simulink model "SimpleEKF_2007a"  (Simulink 6.6)
settings: Solver=FixedStepDiscrete  StartTime=0.0  StopTime=300  FixedStep=0.01  RelTol=1e-3
values from neighbouring files (symbols this model uses):
  initP = diag([ 1 1 1 1e5 1e5 1 1e5 1e5 1e5 ])    [SimpleEKF_init.m.m]
undefined symbols (not defined in the file or in its folder): DiscIntNeverNeededParam, gcbh, hwbcalib_subsystem
libraries: simulink x8, dspmtrx3 x5, dspinverses x1
(part 3 of 9)

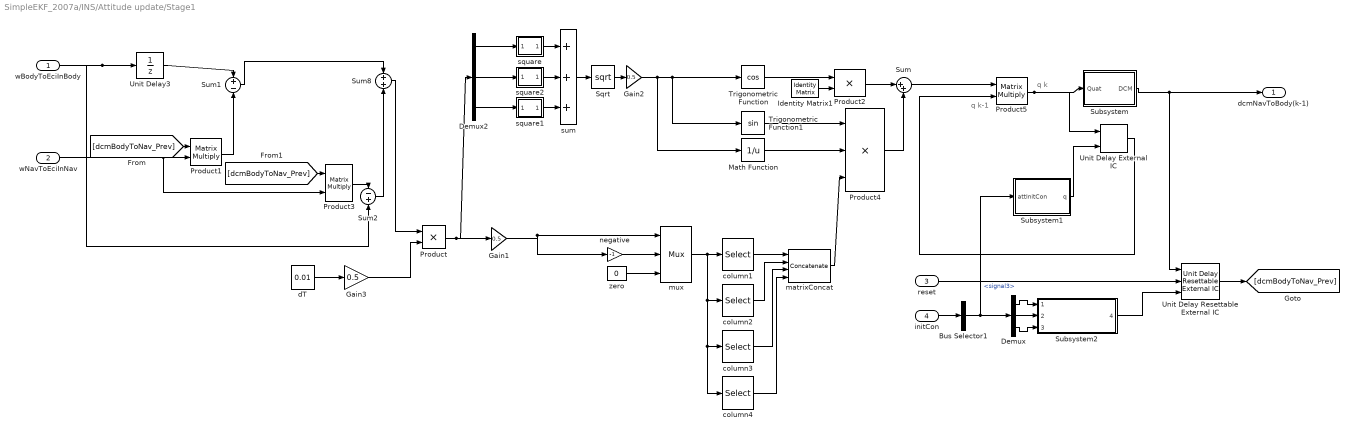
== system SimpleEKF_2007a/INS/Attitude update/Stage1 ==
  note: q k-1
  note: q k
  wBodyToEciInBody : Inport  OutDataType=fixdt(1,16,0)  OutScaling=[]
  wNavToEciInNav : Inport  Port=2  PortDimensions=3  SampleTime=0.01  OutDataType=fixdt(1,16,0)  OutScaling=[]
  reset : Inport  Port=3  PortDimensions=1  SampleTime=0.01  OutDataType=fixdt(1,16,0)  OutScaling=[]
  initCon : Inport  Port=4  OutDataType=fixdt(1,16,0)  OutScaling=[]
  Bus Selector1 : BusSelector  OutputSignals=signal3
  Demux : Demux  Outputs=3
  Demux2 : Demux  Outputs=3
  Gain1 : Gain  Gain=0.5  ParameterDataType=fixdt(1,16,0)  ParameterScaling=[]  OutDataType=fixdt(1,16,0)  OutScaling=[]  SampleTime=0.01
  Gain2 : Gain  Gain=0.5  ParameterDataType=fixdt(1,16,0)  ParameterScaling=[]  OutDataType=fixdt(1,16,0)  OutScaling=[]  SampleTime=0.01
  Gain3 : Gain  Gain=0.5  ParameterDataType=fixdt(1,16,0)  ParameterScaling=[]  OutDataType=fixdt(1,16,0)  OutScaling=[]  SampleTime=0.01
  Identity Matrix1 : dspmtrx3/Identity Matrix  Inherit=off  N=4  Ts=0.01  dataType=double  isSigned=on  wordLen=16  udDataType=sfix(16)  fracBitsMode=Best precision  numFracBits=15
  Math Function : Math  Operator=reciprocal  SampleTime=0.01  OutDataType=fixdt(1,16,0)  OutScaling=[]  SaturateOnIntegerOverflow=on
  Product : Product  OutDataType=fixdt(1,16,0)  OutScaling=[]  RndMeth=Zero
  Product1 : Product  Multiplication=Matrix(*)  OutDataType=fixdt(1,16,0)  OutScaling=[]  SampleTime=0.01  RndMeth=Zero
  Product2 : Product  OutDataType=fixdt(1,16,0)  OutScaling=[]  SampleTime=0.01  RndMeth=Zero
  Product3 : Product  Multiplication=Matrix(*)  OutDataType=fixdt(1,16,0)  OutScaling=[]  SampleTime=0.01  RndMeth=Zero
  Product4 : Product  Inputs=3  OutDataType=fixdt(1,16,0)  OutScaling=[]  SampleTime=0.01  RndMeth=Zero
  Product5 : Product  Multiplication=Matrix(*)  OutDataType=fixdt(1,16,0)  OutScaling=[]  SampleTime=0.01  RndMeth=Zero
  Sqrt : Math  Operator=sqrt  OutDataType=fixdt(1,16,0)  OutScaling=[]  SaturateOnIntegerOverflow=on
  Subsystem : Subsystem
  Subsystem1 : Subsystem
  Subsystem2 : Subsystem
  Sum : Sum  Inputs=|++  OutDataType=fixdt(1,16,0)  OutScaling=[]
  Sum1 : Sum  Inputs=+-  OutDataType=fixdt(1,16,0)  OutScaling=[]  SampleTime=0.01
  Sum2 : Sum  Inputs=-+  OutDataType=fixdt(1,16,0)  OutScaling=[]  SampleTime=0.01
  Sum8 : Sum  OutDataType=fixdt(1,16,0)  OutScaling=[]  SampleTime=0.01
  Trigonometric Function : Trigonometry  Operator=cos  SampleTime=0.01
  Trigonometric Function1 : Trigonometry  SampleTime=0.01
  Unit Delay External IC : simulink/Additional Math & Discrete/Additional Discrete/Unit Delay External IC  SystemSampleTime=-1  tsamp=-1
  Unit Delay Resettable External IC : simulink/Additional Math & Discrete/Additional Discrete/Unit Delay Resettable External IC  SystemSampleTime=-1  tsamp=0.01
  Unit Delay3 : UnitDelay  X0=[0 0 0.]  SampleTime=0.01
  column1 : Selector  Tag=MBDLibrary v2007b.1  IndexOptions=Index vector (dialog)  Indices=[7 1 2 3]  OutputSizes=1  InputPortWidth=7  mask(Mux Selector (MBDLibrary)){InputPortWidth_mbdlib=7, Indices_mbdlib=[7 1 2 3]}
      mask prompts: InputPortWidth_mbdlib "Input Port Width"; Indices_mbdlib "Output Indices"
      mask help: Changes the order of the inputs.
      settings: OpenFcn=|
      | if exist('mbdlib_dialog')
      |    mbdlib_dialog(gcb,'open')
      | else
      |    open_system(gcb, 'mask')
      | end
      settings: CloseFcn=|
      | if exist('mbdlib_selector')
      |    mbdlib_selector(gcb)
      | end
      mask Help: The SELECTOR block is a MULTIPLEXED SELECTOR block, used to change the input/output order of a multiplexed data stream.
      mask Display:
      | port_label('input', 1,'[7]')
      | text(1.0,0.875,'7', 'horizontalAlignment', 'right')
      | text(1.0,0.625,'1', 'horizontalAlignment', 'right')
      | text(1.0,0.375,'2', 'horizontalAlignment', 'right')
      | text(1.0,0.125,'3', 'horizontalAlignment', 'right')
  column2 : Selector  Tag=MBDLibrary v2007b.1  IndexOptions=Index vector (dialog)  Indices=[4 7 6 2]  OutputSizes=1  InputPortWidth=7  mask(Mux Selector (MBDLibrary)){InputPortWidth_mbdlib=7, Indices_mbdlib=[4 7 6 2]}
      mask prompts: InputPortWidth_mbdlib "Input Port Width"; Indices_mbdlib "Output Indices"
      mask help: Changes the order of the inputs.
      settings: OpenFcn=|
      | if exist('mbdlib_dialog')
      |    mbdlib_dialog(gcb,'open')
      | else
      |    open_system(gcb, 'mask')
      | end
      settings: CloseFcn=|
      | if exist('mbdlib_selector')
      |    mbdlib_selector(gcb)
      | end
      mask Help: The SELECTOR block is a MULTIPLEXED SELECTOR block, used to change the input/output order of a multiplexed data stream.
      mask Display:
      | port_label('input', 1,'[7]')
      | text(1.0,0.875,'4', 'horizontalAlignment', 'right')
      | text(1.0,0.625,'7', 'horizontalAlignment', 'right')
      | text(1.0,0.375,'6', 'horizontalAlignment', 'right')
      | text(1.0,0.125,'2', 'horizontalAlignment', 'right')
  column3 : Selector  Tag=MBDLibrary v2007b.1  IndexOptions=Index vector (dialog)  Indices=[5 3 7 4]  OutputSizes=1  InputPortWidth=7  mask(Mux Selector (MBDLibrary)){InputPortWidth_mbdlib=7, Indices_mbdlib=[5 3 7 4]}
      mask prompts: InputPortWidth_mbdlib "Input Port Width"; Indices_mbdlib "Output Indices"
      mask help: Changes the order of the inputs.
      settings: OpenFcn=|
      | if exist('mbdlib_dialog')
      |    mbdlib_dialog(gcb,'open')
      | else
      |    open_system(gcb, 'mask')
      | end
      settings: CloseFcn=|
      | if exist('mbdlib_selector')
      |    mbdlib_selector(gcb)
      | end
      mask Help: The SELECTOR block is a MULTIPLEXED SELECTOR block, used to change the input/output order of a multiplexed data stream.
      mask Display:
      | port_label('input', 1,'[7]')
      | text(1.0,0.875,'5', 'horizontalAlignment', 'right')
      | text(1.0,0.625,'3', 'horizontalAlignment', 'right')
      | text(1.0,0.375,'7', 'horizontalAlignment', 'right')
      | text(1.0,0.125,'4', 'horizontalAlignment', 'right')
  column4 : Selector  Tag=MBDLibrary v2007b.1  IndexOptions=Index vector (dialog)  Indices=[6 5 1 7]  OutputSizes=1  InputPortWidth=7  mask(Mux Selector (MBDLibrary)){InputPortWidth_mbdlib=7, Indices_mbdlib=[6 5 1 7]}
      mask prompts: InputPortWidth_mbdlib "Input Port Width"; Indices_mbdlib "Output Indices"
      mask help: Changes the order of the inputs.
      settings: OpenFcn=|
      | if exist('mbdlib_dialog')
      |    mbdlib_dialog(gcb,'open')
      | else
      |    open_system(gcb, 'mask')
      | end
      settings: CloseFcn=|
      | if exist('mbdlib_selector')
      |    mbdlib_selector(gcb)
      | end
      mask Help: The SELECTOR block is a MULTIPLEXED SELECTOR block, used to change the input/output order of a multiplexed data stream.
      mask Display:
      | port_label('input', 1,'[7]')
      | text(1.0,0.875,'6', 'horizontalAlignment', 'right')
      | text(1.0,0.625,'5', 'horizontalAlignment', 'right')
      | text(1.0,0.375,'1', 'horizontalAlignment', 'right')
      | text(1.0,0.125,'7', 'horizontalAlignment', 'right')
  dT : Constant  Value=0.01  OutDataType=fixdt(1,16,0)  OutScaling=[]
  matrixConcat : Concatenate  Tag=MBDLibrary v2007b.1  NumInputs=4  Mode=Multidimensional array  ConcatenateDimension=2  mask(Matrix Concat (MBDLibrary)){concatDim=Horizontal, numInputs_mbdlib=4}
      mask prompts: concatDim "Type of Concatenate"; numInputs_mbdlib "Number of Inputs"
      mask help: Concatenate input signals of the same data type to create a contiguous output signal.
      settings: OpenFcn=|
      | if exist('mbdlib_dialog')
      |    mbdlib_dialog(gcb,'open')
      | else
      |    open_system(gcb, 'mask')
      | end
      settings: CloseFcn=|
      | if exist('mbdlib_matrixConcatenate')
      |    mbdlib_matrixConcatenate(gcb, 'mask')
      | end
      mask Help:
      | The MATRIX CONCAT block concatenates input signals from the dame data type and creates a contigouos output matrix.
      | In vector mode, all input signals must be either vectors or one-row [1xM] matrices or one-column [Mx1] matrices or a combination of vectors and either one-row matrices or one-column matrices. The output is a vector if all inputs are vectors. The output is a one-row or one-column matrix if any of the inputs are one-row or one-column matrices respectively.
      | 
      | Matrix mode treats vector inputs as one-column matrices. The output is always a matrix.
      mask StyleString: popup(Vertical|Horizontal),edit
      mask Display:
      | plot([0.1 0.3 0.3 0.1 0.1], [0.1 0.1 0.9 0.9 0.1])
      | plot([0.4 0.6 0.6 0.4 0.4], [0.1 0.1 0.9 0.9 0.1])
      | plot([0.7 0.9 0.9 0.7 0.7], [0.1 0.1 0.9 0.9 0.1])
  mux : Mux  Tag=MBDLibrary v2007b.1  Inputs=3  mask(Mux (MBDLibrary)){Inputs_mbdlib=3}
      mask prompts: Inputs_mbdlib "Number of Inputs"
      mask help: Converts multipule inputs to a vector.
      settings: OpenFcn=|
      | if exist('mbdlib_dialog')
      |    mbdlib_dialog(gcb,'open')
      | else
      |    open_system(gcb, 'mask')
      | end
      mask Help: The MUX block provides a vector output to the model for separate inputs.  The output order will correspond to the input order (from the first input at the top of the block to the last input at the bottom of the block).
  negative : Gain  Tag=MBDLibrary v2007b.1  Gain=-1  ParameterDataType=fixdt(1,16,0)  ParameterScaling=[]  OutDataType=fixdt(1,16,0)  OutScaling=[]  RndMeth=Zero  mask(Gain (MBDLibrary)){gain_mbdlib=-1}
      mask prompts: gain_mbdlib "Gain"
      mask help: Multiplies the input by the gain.
      settings: OpenFcn=|
      | if exist('mbdlib_dialog')
      |    mbdlib_dialog(gcb,'open')
      | else
      |    open_system(gcb, 'mask')
      | end
      mask Help: The GAIN block multiplies the input by the gain value.  This block may accept any data types other than boolean.  The user must take care to not use a non-integer gain for int32/uint32 inputs.
      mask Display: disp([get_param(gcb, 'Gain') 'x'])
  square : Subsystem  Tag=MBDLibrary v2007b.1
      settings: OpenFcn=|
      | if exist('mbdlib_dialog')
      |    mbdlib_dialog(gcb,'open')
      | else
      |    open_system(gcb, 'mask')
      | end
      mask Type: Square (MBDLibrary)
      mask Description: Squares the input.
      mask Help: file:///c:\Program Files\MATLAB\R2007b\toolbox\Guidance_and_Navigation_Global\help_files\GeneralUtilities\MBDLibrary\mathfunctions\square.html
      mask Display: disp('x^2', 'texmode', 'on')
  square1 : Subsystem  Tag=MBDLibrary v2007b.1
      settings: OpenFcn=|
      | if exist('mbdlib_dialog')
      |    mbdlib_dialog(gcb,'open')
      | else
      |    open_system(gcb, 'mask')
      | end
      mask Type: Square (MBDLibrary)
      mask Description: Squares the input.
      mask Help: file:///c:\Program Files\MATLAB\R2007b\toolbox\Guidance_and_Navigation_Global\help_files\GeneralUtilities\MBDLibrary\mathfunctions\square.html
      mask Display: disp('x^2', 'texmode', 'on')
  square2 : Subsystem  Tag=MBDLibrary v2007b.1
      settings: OpenFcn=|
      | if exist('mbdlib_dialog')
      |    mbdlib_dialog(gcb,'open')
      | else
      |    open_system(gcb, 'mask')
      | end
      mask Type: Square (MBDLibrary)
      mask Description: Squares the input.
      mask Help: file:///c:\Program Files\MATLAB\R2007b\toolbox\Guidance_and_Navigation_Global\help_files\GeneralUtilities\MBDLibrary\mathfunctions\square.html
      mask Display: disp('x^2', 'texmode', 'on')
  sum : Sum  Tag=MBDLibrary v2007b.1  Inputs=+++  OutDataType=fixdt(1,16,0)  OutScaling=[]  RndMeth=Zero  InputSameDT=on  mask(Sum (MBDLibrary)){inputs_mbdlib=+++}
      mask prompts: inputs_mbdlib "List of signs"
      mask help: Adds values together.
      settings: OpenFcn=|
      | if exist('mbdlib_dialog')
      |    mbdlib_dialog(gcb,'open')
      | else
      |    open_system(gcb, 'mask')
      | end
      mask Help: file:///c:\Program Files\MATLAB\R2007b\toolbox\Guidance_and_Navigation_Global\help_files\GeneralUtilities\MBDLibrary\mathfunctions\sum.html
  zero : Constant  Tag=MBDLibrary v2007b.1  Value=0  VectorParams1D=off  OutDataType=fixdt(1,16,0)  OutScaling=[]  mask(Constant (MBDLibrary)){Value_mbdlib=0, OutDataTypeMode_mbdlib=double}
      mask prompts: Value_mbdlib "Constant"; OutDataTypeMode_mbdlib "Data Type"
      mask help: Outputs a constant value
      settings: AttributesFormatString={%<OutDataTypeMode>}
      settings: OpenFcn=|
      | if exist('mbdlib_dialog')
      |    mbdlib_dialog(gcb,'open')
      | else
      |    open_system(gcb, 'mask')
      | end
      settings: CloseFcn=|
      | if exist('mbdlib_dialog')
      |    mbdlib_constant(gcb)
      | end
      mask Help: The CONSTANT block outputs a constant value to the system.
      mask StyleString: edit,popup(double|single|boolean|int32|uint32)
  dcmNavToBody(k-1) : Outport  OutDataType=fixdt(1,16,0)  OutScaling=[]
  wires:
  wBodyToEciInBody/1 -> Sum2/2, Unit Delay3/1
  wNavToEciInNav/1 -> Product1/2, Product3/2
  Demux2/3 -> square1/1(squareLibIn)
  Subsystem/1(DCM) -> dcmNavToBody(k-1)/1, Unit Delay Resettable External IC/1
  Demux2/2 -> square2/1(squareLibIn)
  Unit Delay External IC/1 -> Product5/2
  Product5/1 -> Unit Delay External IC/1, Subsystem/1(Quat)
  Sum/1 -> Product5/1
  Product4/1 -> Sum/2
  Product2/1 -> Sum/1
  Identity Matrix1/1 -> Product2/2
  Trigonometric Function/1 -> Product2/1
  Gain2/1 -> Math Function/1, Trigonometric Function/1, Trigonometric Function1/1
  Sqrt/1 -> Gain2/1
  sum/1 -> Sqrt/1
  square1/1(squareLibOut) -> sum/3
  square2/1(squareLibOut) -> sum/2
  square/1(squareLibOut) -> sum/1
  Demux2/1 -> square/1(squareLibIn)
  column4/1 -> matrixConcat/4
  Gain1/1 -> mux/1, negative/1
  mux/1 -> column2/1, column3/1, column4/1, column1/1
  column1/1 -> matrixConcat/1
  column2/1 -> matrixConcat/2
  column3/1 -> matrixConcat/3
  negative/1 -> mux/2
  zero/1 -> mux/3
  Sum1/1 -> Sum8/1
  Sum2/1 -> Sum8/2
  Product3/1 -> Sum2/1
  Unit Delay3/1 -> Sum1/1
  Product1/1 -> Sum1/2
  dT/1 -> Gain3/1
  Sum8/1 -> Product/1
  Gain3/1 -> Product/2
  Product/1 -> Gain1/1, Demux2/1
  [dcmBodyToNav_Prev] -> Product1/1
  [dcmBodyToNav_Prev] -> Product3/1
  Trigonometric Function1/1 -> Product4/1
  Math Function/1 -> Product4/2
  matrixConcat/1 -> Product4/3
  Subsystem1/1(q) -> Unit Delay External IC/2
  reset/1 -> Unit Delay Resettable External IC/2
  initCon/1 -> Bus Selector1/1
  Bus Selector1/1 -> Demux/1, Subsystem1/1(attInitCon)  "<signal3>"
  Demux/1 -> Subsystem2/1(1)
  Demux/2 -> Subsystem2/2(2)
  Demux/3 -> Subsystem2/3(3)
  Unit Delay Resettable External IC/1 -> [dcmBodyToNav_Prev]
  Subsystem2/1(4) -> Unit Delay Resettable External IC/3

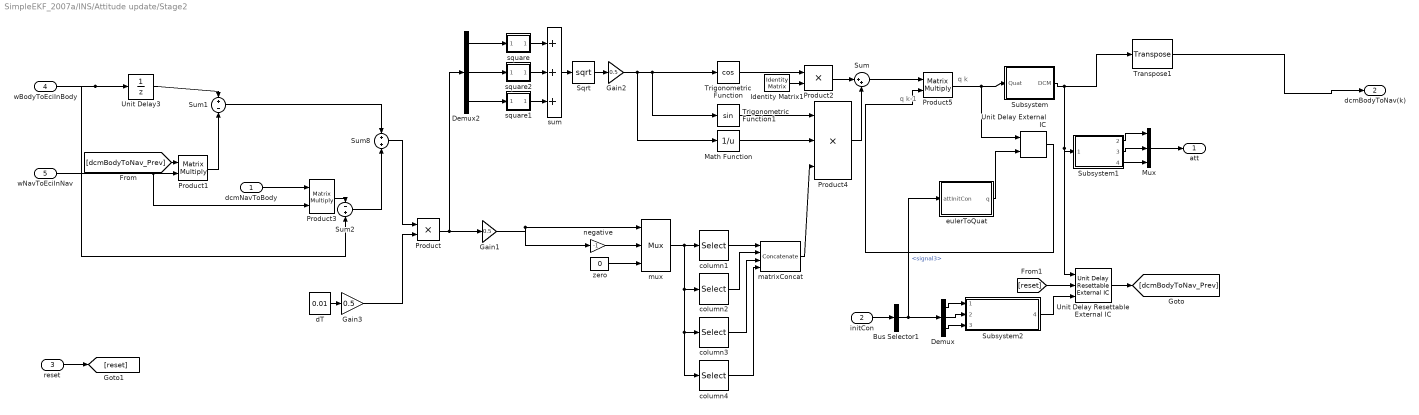
== system SimpleEKF_2007a/INS/Attitude update/Stage2 ==
  note: q k-1
  note: q k
  dcmNavToBody : Inport  PortDimensions=[3,3]  SampleTime=0.01  OutDataType=fixdt(1,16,0)  OutScaling=[]
  initCon : Inport  Port=2  OutDataType=fixdt(1,16,0)  OutScaling=[]
  reset : Inport  Port=3  PortDimensions=1  SampleTime=0.01  OutDataType=fixdt(1,16,0)  OutScaling=[]
  wBodyToEciInBody : Inport  Port=4  PortDimensions=3  SampleTime=0.01  OutDataType=fixdt(1,16,0)  OutScaling=[]
  wNavToEciInNav : Inport  Port=5  PortDimensions=3  SampleTime=0.01  OutDataType=fixdt(1,16,0)  OutScaling=[]
  Bus Selector1 : BusSelector  OutputSignals=signal3
  Demux : Demux  Outputs=3
  Demux2 : Demux  Outputs=3
  Gain1 : Gain  Gain=0.5  ParameterDataType=fixdt(1,16,0)  ParameterScaling=[]  OutDataType=fixdt(1,16,0)  OutScaling=[]  SampleTime=0.01
  Gain2 : Gain  Gain=0.5  ParameterDataType=fixdt(1,16,0)  ParameterScaling=[]  OutDataType=fixdt(1,16,0)  OutScaling=[]  SampleTime=0.01
  Gain3 : Gain  Gain=0.5  ParameterDataType=fixdt(1,16,0)  ParameterScaling=[]  OutDataType=fixdt(1,16,0)  OutScaling=[]  SampleTime=0.01
  Identity Matrix1 : dspmtrx3/Identity Matrix  Inherit=off  N=4  Ts=0.01  dataType=double  isSigned=on  wordLen=16  udDataType=sfix(16)  fracBitsMode=Best precision  numFracBits=15
  Math Function : Math  Operator=reciprocal  SampleTime=0.01  OutDataType=fixdt(1,16,0)  OutScaling=[]  SaturateOnIntegerOverflow=on
  Mux : Mux  Inputs=3
  Product : Product  OutDataType=fixdt(1,16,0)  OutScaling=[]  RndMeth=Zero
  Product1 : Product  Multiplication=Matrix(*)  OutDataType=fixdt(1,16,0)  OutScaling=[]  SampleTime=0.01  RndMeth=Zero
  Product2 : Product  OutDataType=fixdt(1,16,0)  OutScaling=[]  SampleTime=0.01  RndMeth=Zero
  Product3 : Product  Multiplication=Matrix(*)  OutDataType=fixdt(1,16,0)  OutScaling=[]  SampleTime=0.01  RndMeth=Zero
  Product4 : Product  Inputs=3  OutDataType=fixdt(1,16,0)  OutScaling=[]  SampleTime=0.01  RndMeth=Zero
  Product5 : Product  Multiplication=Matrix(*)  OutDataType=fixdt(1,16,0)  OutScaling=[]  SampleTime=0.01  RndMeth=Zero
  Sqrt : Math  Operator=sqrt  OutDataType=fixdt(1,16,0)  OutScaling=[]  SaturateOnIntegerOverflow=on
  Subsystem : Subsystem
  Subsystem1 : Subsystem
  Subsystem2 : Subsystem
  Sum : Sum  Inputs=|++  OutDataType=fixdt(1,16,0)  OutScaling=[]
  Sum1 : Sum  Inputs=+-  OutDataType=fixdt(1,16,0)  OutScaling=[]  SampleTime=0.01
  Sum2 : Sum  Inputs=-+  OutDataType=fixdt(1,16,0)  OutScaling=[]  SampleTime=0.01
  Sum8 : Sum  OutDataType=fixdt(1,16,0)  OutScaling=[]  SampleTime=0.01
  Transpose1 : dspmtrx3/Transpose  SystemSampleTime=-1  Hermitian=off  overflowFlag=off
  Trigonometric Function : Trigonometry  Operator=cos  SampleTime=0.01
  Trigonometric Function1 : Trigonometry  SampleTime=0.01
  Unit Delay External IC : simulink/Additional Math & Discrete/Additional Discrete/Unit Delay External IC  SystemSampleTime=-1  tsamp=-1
  Unit Delay Resettable External IC : simulink/Additional Math & Discrete/Additional Discrete/Unit Delay Resettable External IC  SystemSampleTime=-1  tsamp=0.01
  Unit Delay3 : UnitDelay  X0=[0 0 0]  SampleTime=0.01
  column1 : Selector  Tag=MBDLibrary v2007b.1  IndexOptions=Index vector (dialog)  Indices=[7 1 2 3]  OutputSizes=1  InputPortWidth=7  mask(Mux Selector (MBDLibrary)){InputPortWidth_mbdlib=7, Indices_mbdlib=[7 1 2 3]}
      mask prompts: InputPortWidth_mbdlib "Input Port Width"; Indices_mbdlib "Output Indices"
      mask help: Changes the order of the inputs.
      settings: OpenFcn=|
      | if exist('mbdlib_dialog')
      |    mbdlib_dialog(gcb,'open')
      | else
      |    open_system(gcb, 'mask')
      | end
      settings: CloseFcn=|
      | if exist('mbdlib_selector')
      |    mbdlib_selector(gcb)
      | end
      mask Help: The SELECTOR block is a MULTIPLEXED SELECTOR block, used to change the input/output order of a multiplexed data stream.
      mask Display:
      | port_label('input', 1,'[7]')
      | text(1.0,0.875,'7', 'horizontalAlignment', 'right')
      | text(1.0,0.625,'1', 'horizontalAlignment', 'right')
      | text(1.0,0.375,'2', 'horizontalAlignment', 'right')
      | text(1.0,0.125,'3', 'horizontalAlignment', 'right')
  column2 : Selector  Tag=MBDLibrary v2007b.1  IndexOptions=Index vector (dialog)  Indices=[4 7 6 2]  OutputSizes=1  InputPortWidth=7  mask(Mux Selector (MBDLibrary)){InputPortWidth_mbdlib=7, Indices_mbdlib=[4 7 6 2]}
      mask prompts: InputPortWidth_mbdlib "Input Port Width"; Indices_mbdlib "Output Indices"
      mask help: Changes the order of the inputs.
      settings: OpenFcn=|
      | if exist('mbdlib_dialog')
      |    mbdlib_dialog(gcb,'open')
      | else
      |    open_system(gcb, 'mask')
      | end
      settings: CloseFcn=|
      | if exist('mbdlib_selector')
      |    mbdlib_selector(gcb)
      | end
      mask Help: The SELECTOR block is a MULTIPLEXED SELECTOR block, used to change the input/output order of a multiplexed data stream.
      mask Display:
      | port_label('input', 1,'[7]')
      | text(1.0,0.875,'4', 'horizontalAlignment', 'right')
      | text(1.0,0.625,'7', 'horizontalAlignment', 'right')
      | text(1.0,0.375,'6', 'horizontalAlignment', 'right')
      | text(1.0,0.125,'2', 'horizontalAlignment', 'right')
  column3 : Selector  Tag=MBDLibrary v2007b.1  IndexOptions=Index vector (dialog)  Indices=[5 3 7 4]  OutputSizes=1  InputPortWidth=7  mask(Mux Selector (MBDLibrary)){InputPortWidth_mbdlib=7, Indices_mbdlib=[5 3 7 4]}
      mask prompts: InputPortWidth_mbdlib "Input Port Width"; Indices_mbdlib "Output Indices"
      mask help: Changes the order of the inputs.
      settings: OpenFcn=|
      | if exist('mbdlib_dialog')
      |    mbdlib_dialog(gcb,'open')
      | else
      |    open_system(gcb, 'mask')
      | end
      settings: CloseFcn=|
      | if exist('mbdlib_selector')
      |    mbdlib_selector(gcb)
      | end
      mask Help: The SELECTOR block is a MULTIPLEXED SELECTOR block, used to change the input/output order of a multiplexed data stream.
      mask Display:
      | port_label('input', 1,'[7]')
      | text(1.0,0.875,'5', 'horizontalAlignment', 'right')
      | text(1.0,0.625,'3', 'horizontalAlignment', 'right')
      | text(1.0,0.375,'7', 'horizontalAlignment', 'right')
      | text(1.0,0.125,'4', 'horizontalAlignment', 'right')
  column4 : Selector  Tag=MBDLibrary v2007b.1  IndexOptions=Index vector (dialog)  Indices=[6 5 1 7]  OutputSizes=1  InputPortWidth=7  mask(Mux Selector (MBDLibrary)){InputPortWidth_mbdlib=7, Indices_mbdlib=[6 5 1 7]}
      mask prompts: InputPortWidth_mbdlib "Input Port Width"; Indices_mbdlib "Output Indices"
      mask help: Changes the order of the inputs.
      settings: OpenFcn=|
      | if exist('mbdlib_dialog')
      |    mbdlib_dialog(gcb,'open')
      | else
      |    open_system(gcb, 'mask')
      | end
      settings: CloseFcn=|
      | if exist('mbdlib_selector')
      |    mbdlib_selector(gcb)
      | end
      mask Help: The SELECTOR block is a MULTIPLEXED SELECTOR block, used to change the input/output order of a multiplexed data stream.
      mask Display:
      | port_label('input', 1,'[7]')
      | text(1.0,0.875,'6', 'horizontalAlignment', 'right')
      | text(1.0,0.625,'5', 'horizontalAlignment', 'right')
      | text(1.0,0.375,'1', 'horizontalAlignment', 'right')
      | text(1.0,0.125,'7', 'horizontalAlignment', 'right')
  dT : Constant  Value=0.01  OutDataType=fixdt(1,16,0)  OutScaling=[]
  eulerToQuat : Subsystem
  matrixConcat : Concatenate  Tag=MBDLibrary v2007b.1  NumInputs=4  Mode=Multidimensional array  ConcatenateDimension=2  mask(Matrix Concat (MBDLibrary)){concatDim=Horizontal, numInputs_mbdlib=4}
      mask prompts: concatDim "Type of Concatenate"; numInputs_mbdlib "Number of Inputs"
      mask help: Concatenate input signals of the same data type to create a contiguous output signal.
      settings: OpenFcn=|
      | if exist('mbdlib_dialog')
      |    mbdlib_dialog(gcb,'open')
      | else
      |    open_system(gcb, 'mask')
      | end
      settings: CloseFcn=|
      | if exist('mbdlib_matrixConcatenate')
      |    mbdlib_matrixConcatenate(gcb, 'mask')
      | end
      mask Help:
      | The MATRIX CONCAT block concatenates input signals from the dame data type and creates a contigouos output matrix.
      | In vector mode, all input signals must be either vectors or one-row [1xM] matrices or one-column [Mx1] matrices or a combination of vectors and either one-row matrices or one-column matrices. The output is a vector if all inputs are vectors. The output is a one-row or one-column matrix if any of the inputs are one-row or one-column matrices respectively.
      | 
      | Matrix mode treats vector inputs as one-column matrices. The output is always a matrix.
      mask StyleString: popup(Vertical|Horizontal),edit
      mask Display:
      | plot([0.1 0.3 0.3 0.1 0.1], [0.1 0.1 0.9 0.9 0.1])
      | plot([0.4 0.6 0.6 0.4 0.4], [0.1 0.1 0.9 0.9 0.1])
      | plot([0.7 0.9 0.9 0.7 0.7], [0.1 0.1 0.9 0.9 0.1])
  mux : Mux  Tag=MBDLibrary v2007b.1  Inputs=3  mask(Mux (MBDLibrary)){Inputs_mbdlib=3}
      mask prompts: Inputs_mbdlib "Number of Inputs"
      mask help: Converts multipule inputs to a vector.
      settings: OpenFcn=|
      | if exist('mbdlib_dialog')
      |    mbdlib_dialog(gcb,'open')
      | else
      |    open_system(gcb, 'mask')
      | end
      mask Help: The MUX block provides a vector output to the model for separate inputs.  The output order will correspond to the input order (from the first input at the top of the block to the last input at the bottom of the block).
  negative : Gain  Tag=MBDLibrary v2007b.1  Gain=-1  ParameterDataType=fixdt(1,16,0)  ParameterScaling=[]  OutDataType=fixdt(1,16,0)  OutScaling=[]  RndMeth=Zero  mask(Gain (MBDLibrary)){gain_mbdlib=-1}
      mask prompts: gain_mbdlib "Gain"
      mask help: Multiplies the input by the gain.
      settings: OpenFcn=|
      | if exist('mbdlib_dialog')
      |    mbdlib_dialog(gcb,'open')
      | else
      |    open_system(gcb, 'mask')
      | end
      mask Help: The GAIN block multiplies the input by the gain value.  This block may accept any data types other than boolean.  The user must take care to not use a non-integer gain for int32/uint32 inputs.
      mask Display: disp([get_param(gcb, 'Gain') 'x'])
  square : Subsystem  Tag=MBDLibrary v2007b.1
      settings: OpenFcn=|
      | if exist('mbdlib_dialog')
      |    mbdlib_dialog(gcb,'open')
      | else
      |    open_system(gcb, 'mask')
      | end
      mask Type: Square (MBDLibrary)
      mask Description: Squares the input.
      mask Help: file:///c:\Program Files\MATLAB\R2007b\toolbox\Guidance_and_Navigation_Global\help_files\GeneralUtilities\MBDLibrary\mathfunctions\square.html
      mask Display: disp('x^2', 'texmode', 'on')
  square1 : Subsystem  Tag=MBDLibrary v2007b.1
      settings: OpenFcn=|
      | if exist('mbdlib_dialog')
      |    mbdlib_dialog(gcb,'open')
      | else
      |    open_system(gcb, 'mask')
      | end
      mask Type: Square (MBDLibrary)
      mask Description: Squares the input.
      mask Help: file:///c:\Program Files\MATLAB\R2007b\toolbox\Guidance_and_Navigation_Global\help_files\GeneralUtilities\MBDLibrary\mathfunctions\square.html
      mask Display: disp('x^2', 'texmode', 'on')
  square2 : Subsystem  Tag=MBDLibrary v2007b.1
      settings: OpenFcn=|
      | if exist('mbdlib_dialog')
      |    mbdlib_dialog(gcb,'open')
      | else
      |    open_system(gcb, 'mask')
      | end
      mask Type: Square (MBDLibrary)
      mask Description: Squares the input.
      mask Help: file:///c:\Program Files\MATLAB\R2007b\toolbox\Guidance_and_Navigation_Global\help_files\GeneralUtilities\MBDLibrary\mathfunctions\square.html
      mask Display: disp('x^2', 'texmode', 'on')
  sum : Sum  Tag=MBDLibrary v2007b.1  Inputs=+++  OutDataType=fixdt(1,16,0)  OutScaling=[]  RndMeth=Zero  InputSameDT=on  mask(Sum (MBDLibrary)){inputs_mbdlib=+++}
      mask prompts: inputs_mbdlib "List of signs"
      mask help: Adds values together.
      settings: OpenFcn=|
      | if exist('mbdlib_dialog')
      |    mbdlib_dialog(gcb,'open')
      | else
      |    open_system(gcb, 'mask')
      | end
      mask Help: file:///c:\Program Files\MATLAB\R2007b\toolbox\Guidance_and_Navigation_Global\help_files\GeneralUtilities\MBDLibrary\mathfunctions\sum.html
  zero : Constant  Tag=MBDLibrary v2007b.1  Value=0  VectorParams1D=off  OutDataType=fixdt(1,16,0)  OutScaling=[]  mask(Constant (MBDLibrary)){Value_mbdlib=0, OutDataTypeMode_mbdlib=double}
      mask prompts: Value_mbdlib "Constant"; OutDataTypeMode_mbdlib "Data Type"
      mask help: Outputs a constant value
      settings: AttributesFormatString={%<OutDataTypeMode>}
      settings: OpenFcn=|
      | if exist('mbdlib_dialog')
      |    mbdlib_dialog(gcb,'open')
      | else
      |    open_system(gcb, 'mask')
      | end
      settings: CloseFcn=|
      | if exist('mbdlib_dialog')
      |    mbdlib_constant(gcb)
      | end
      mask Help: The CONSTANT block outputs a constant value to the system.
      mask StyleString: edit,popup(double|single|boolean|int32|uint32)
  att : Outport  PortDimensions=3  SampleTime=0.01  OutDataType=fixdt(1,16,0)  OutScaling=[]
  dcmBodyToNav(k) : Outport  Port=2  OutDataType=fixdt(1,16,0)  OutScaling=[]
  wires:
  wBodyToEciInBody/1 -> Sum2/2, Unit Delay3/1
  wNavToEciInNav/1 -> Product1/2, Product3/2
  Demux2/3 -> square1/1(squareLibIn)
  Subsystem/1(DCM) -> Unit Delay Resettable External IC/1, Subsystem1/1(1), Transpose1/1
  Demux2/2 -> square2/1(squareLibIn)
  Product5/1 -> Unit Delay External IC/1, Subsystem/1(Quat)
  Sum/1 -> Product5/1
  Product4/1 -> Sum/2
  Product2/1 -> Sum/1
  Identity Matrix1/1 -> Product2/2
  Trigonometric Function/1 -> Product2/1
  Gain2/1 -> Math Function/1, Trigonometric Function/1, Trigonometric Function1/1
  Sqrt/1 -> Gain2/1
  sum/1 -> Sqrt/1
  square1/1(squareLibOut) -> sum/3
  square2/1(squareLibOut) -> sum/2
  square/1(squareLibOut) -> sum/1
  Demux2/1 -> square/1(squareLibIn)
  column4/1 -> matrixConcat/4
  Gain1/1 -> mux/1, negative/1
  mux/1 -> column2/1, column3/1, column4/1, column1/1
  column1/1 -> matrixConcat/1
  column2/1 -> matrixConcat/2
  column3/1 -> matrixConcat/3
  negative/1 -> mux/2
  zero/1 -> mux/3
  Sum1/1 -> Sum8/1
  Sum2/1 -> Sum8/2
  Product3/1 -> Sum2/1
  Unit Delay3/1 -> Sum1/1
  Product1/1 -> Sum1/2
  dT/1 -> Gain3/1
  Sum8/1 -> Product/1
  Gain3/1 -> Product/2
  Product/1 -> Gain1/1, Demux2/1
  [dcmBodyToNav_Prev] -> Product1/1
  Trigonometric Function1/1 -> Product4/1
  Math Function/1 -> Product4/2
  dcmNavToBody/1 -> Product3/1
  Subsystem1/1(2) -> Mux/1
  Subsystem1/2(3) -> Mux/2
  Subsystem1/3(4) -> Mux/3
  matrixConcat/1 -> Product4/3
  Unit Delay Resettable External IC/1 -> [dcmBodyToNav_Prev]
  initCon/1 -> Bus Selector1/1
  Bus Selector1/1 -> Demux/1, eulerToQuat/1(attInitCon)  "<signal3>"
  Demux/1 -> Subsystem2/1(1)
  Demux/2 -> Subsystem2/2(2)
  Demux/3 -> Subsystem2/3(3)
  Unit Delay External IC/1 -> Product5/2
  eulerToQuat/1(q) -> Unit Delay External IC/2
  reset/1 -> [reset]
  [reset] -> Unit Delay Resettable External IC/2
  Subsystem2/1(4) -> Unit Delay Resettable External IC/3
  Transpose1/1 -> dcmBodyToNav(k)/1
  Mux/1 -> att/1

== system SimpleEKF_2007a/INS/Coriolis correction/RM ==
  pos_lat : Inport  PortDimensions=1  SampleTime=0.01  OutDataType=fixdt(1,16,0)  OutScaling=[]
  Constant : Constant  OutDataType=fixdt(1,16,0)  OutScaling=[]
  Constant1 : Constant  Value=1.5  OutDataType=fixdt(1,16,0)  OutScaling=[]
  Math Function : Math  Operator=pow  OutDataType=fixdt(1,16,0)  OutScaling=[]  SaturateOnIntegerOverflow=on
  Product : Product  OutDataType=fixdt(1,16,0)  OutScaling=[]  RndMeth=Zero
  Product1 : Product  OutDataType=fixdt(1,16,0)  OutScaling=[]  RndMeth=Zero
  Sum : Sum  Inputs=|+-  OutDataType=fixdt(1,16,0)  OutScaling=[]
  Sum1 : Sum  Inputs=|+-  OutDataType=fixdt(1,16,0)  OutScaling=[]
  Trigonometric Function : Trigonometry
  constant : Constant  Tag=MBDLibrary v2007b.1  VectorParams1D=off  OutDataType=fixdt(1,16,0)  OutScaling=[]  mask(Constant (MBDLibrary)){Value_mbdlib=1, OutDataTypeMode_mbdlib=double}
      mask prompts: Value_mbdlib "Constant"; OutDataTypeMode_mbdlib "Data Type"
      mask help: Outputs a constant value
      settings: AttributesFormatString={%<OutDataTypeMode>}
      settings: OpenFcn=|
      | if exist('mbdlib_dialog')
      |    mbdlib_dialog(gcb,'open')
      | else
      |    open_system(gcb, 'mask')
      | end
      settings: CloseFcn=|
      | if exist('mbdlib_dialog')
      |    mbdlib_constant(gcb)
      | end
      mask Help: file:///c:\Program Files\MATLAB\R2007b\toolbox\Guidance_and_Navigation_Global\help_files\GeneralUtilities\MBDLibrary\mathfunctions\constant.html
      mask StyleString: edit,popup(double|single|boolean|int32|uint32)
  divide : Product  Tag=MBDLibrary v2007b.1  Inputs=*/  OutDataType=fixdt(1,16,0)  OutScaling=[]  RndMeth=Zero  InputSameDT=on
      settings: OpenFcn=|
      | if exist('mbdlib_dialog')
      |    mbdlib_dialog(gcb,'open')
      | else
      |    open_system(gcb, 'mask')
      | end
      mask Type: Divide (MBDLibrary)
      mask Description: Divides two inputs.
      mask Help: file:///c:\Program Files\MATLAB\R2007b\toolbox\Guidance_and_Navigation_Global\help_files\GeneralUtilities\MBDLibrary\mathfunctions\divide.html
      mask Display:
      | port_label('input',1,'n')
      | port_label('input',2,'d')
      | port_label('output',1,'n/d')
  epsilon : Constant  Value=0.0818191908426  OutDataType=fixdt(1,16,0)  OutScaling=[]
  re : Constant  Value=6378137  OutDataType=fixdt(1,16,0)  OutScaling=[]
  square : Subsystem  Tag=MBDLibrary v2007b.1
      settings: OpenFcn=|
      | if exist('mbdlib_dialog')
      |    mbdlib_dialog(gcb,'open')
      | else
      |    open_system(gcb, 'mask')
      | end
      mask Type: Square (MBDLibrary)
      mask Description: Squares the input.
      mask Help: file:///c:\Program Files\MATLAB\R2007b\toolbox\Guidance_and_Navigation_Global\help_files\GeneralUtilities\MBDLibrary\mathfunctions\square.html
      mask Display: disp('x^2', 'texmode', 'on')
  square1 : Subsystem  Tag=MBDLibrary v2007b.1
      settings: OpenFcn=|
      | if exist('mbdlib_dialog')
      |    mbdlib_dialog(gcb,'open')
      | else
      |    open_system(gcb, 'mask')
      | end
      mask Type: Square (MBDLibrary)
      mask Description: Squares the input.
      mask Help: file:///c:\Program Files\MATLAB\R2007b\toolbox\Guidance_and_Navigation_Global\help_files\GeneralUtilities\MBDLibrary\mathfunctions\square.html
      mask Display: disp('x^2', 'texmode', 'on')
  rm : Outport  PortDimensions=1  SampleTime=0.01  OutDataType=fixdt(1,16,0)  OutScaling=[]
  wires:
  constant/1 -> Sum/1
  epsilon/1 -> square1/1(squareLibIn)
  square1/1(squareLibOut) -> Product/1, Sum1/2
  pos_lat/1 -> Trigonometric Function/1
  Trigonometric Function/1 -> square/1(squareLibIn)
  square/1(squareLibOut) -> Product/2
  Product/1 -> Sum/2
  Sum/1 -> Math Function/1
  divide/1 -> rm/1
  Constant/1 -> Sum1/1
  Constant1/1 -> Math Function/2
  Math Function/1 -> divide/2
  re/1 -> Product1/1
  Sum1/1 -> Product1/2
  Product1/1 -> divide/1

== system SimpleEKF_2007a/INS/Coriolis correction/RN ==
  pos_lat : Inport  PortDimensions=1  SampleTime=0.01  OutDataType=fixdt(1,16,0)  OutScaling=[]
  Product : Product  OutDataType=fixdt(1,16,0)  OutScaling=[]  RndMeth=Zero
  Sqrt : Math  Operator=sqrt  OutDataType=fixdt(1,16,0)  OutScaling=[]  SaturateOnIntegerOverflow=on
  Sum : Sum  Inputs=|+-  OutDataType=fixdt(1,16,0)  OutScaling=[]
  Trigonometric Function : Trigonometry
  constant : Constant  Tag=MBDLibrary v2007b.1  VectorParams1D=off  OutDataType=fixdt(1,16,0)  OutScaling=[]  mask(Constant (MBDLibrary)){Value_mbdlib=1, OutDataTypeMode_mbdlib=double}
      mask prompts: Value_mbdlib "Constant"; OutDataTypeMode_mbdlib "Data Type"
      mask help: Outputs a constant value
      settings: AttributesFormatString={%<OutDataTypeMode>}
      settings: OpenFcn=|
      | if exist('mbdlib_dialog')
      |    mbdlib_dialog(gcb,'open')
      | else
      |    open_system(gcb, 'mask')
      | end
      settings: CloseFcn=|
      | if exist('mbdlib_dialog')
      |    mbdlib_constant(gcb)
      | end
      mask Help: file:///c:\Program Files\MATLAB\R2007b\toolbox\Guidance_and_Navigation_Global\help_files\GeneralUtilities\MBDLibrary\mathfunctions\constant.html
      mask StyleString: edit,popup(double|single|boolean|int32|uint32)
  divide : Product  Tag=MBDLibrary v2007b.1  Inputs=*/  OutDataType=fixdt(1,16,0)  OutScaling=[]  RndMeth=Zero  InputSameDT=on
      settings: OpenFcn=|
      | if exist('mbdlib_dialog')
      |    mbdlib_dialog(gcb,'open')
      | else
      |    open_system(gcb, 'mask')
      | end
      mask Type: Divide (MBDLibrary)
      mask Description: Divides two inputs.
      mask Help: file:///c:\Program Files\MATLAB\R2007b\toolbox\Guidance_and_Navigation_Global\help_files\GeneralUtilities\MBDLibrary\mathfunctions\divide.html
      mask Display:
      | port_label('input',1,'n')
      | port_label('input',2,'d')
      | port_label('output',1,'n/d')
  epsilon : Constant  Value=0.0818191908426  OutDataType=fixdt(1,16,0)  OutScaling=[]
  re : Constant  Value=6378137  OutDataType=fixdt(1,16,0)  OutScaling=[]
  square : Subsystem  Tag=MBDLibrary v2007b.1
      settings: OpenFcn=|
      | if exist('mbdlib_dialog')
      |    mbdlib_dialog(gcb,'open')
      | else
      |    open_system(gcb, 'mask')
      | end
      mask Type: Square (MBDLibrary)
      mask Description: Squares the input.
      mask Help: file:///c:\Program Files\MATLAB\R2007b\toolbox\Guidance_and_Navigation_Global\help_files\GeneralUtilities\MBDLibrary\mathfunctions\square.html
      mask Display: disp('x^2', 'texmode', 'on')
  square1 : Subsystem  Tag=MBDLibrary v2007b.1
      settings: OpenFcn=|
      | if exist('mbdlib_dialog')
      |    mbdlib_dialog(gcb,'open')
      | else
      |    open_system(gcb, 'mask')
      | end
      mask Type: Square (MBDLibrary)
      mask Description: Squares the input.
      mask Help: file:///c:\Program Files\MATLAB\R2007b\toolbox\Guidance_and_Navigation_Global\help_files\GeneralUtilities\MBDLibrary\mathfunctions\square.html
      mask Display: disp('x^2', 'texmode', 'on')
  rn : Outport  PortDimensions=1  SampleTime=0.01  OutDataType=fixdt(1,16,0)  OutScaling=[]
  wires:
  re/1 -> divide/1
  constant/1 -> Sum/1
  epsilon/1 -> square1/1(squareLibIn)
  square1/1(squareLibOut) -> Product/1
  pos_lat/1 -> Trigonometric Function/1
  Trigonometric Function/1 -> square/1(squareLibIn)
  square/1(squareLibOut) -> Product/2
  Product/1 -> Sum/2
  Sum/1 -> Sqrt/1
  Sqrt/1 -> divide/2
  divide/1 -> rn/1

== system SimpleEKF_2007a/INS/Coriolis correction/skewSymmetric ==
  skewLibIn : Inport  OutDataType=fixdt(1,16,0)  OutScaling=[]
  column1 : Selector  Tag=MBDLibrary v2007b.1  IndexOptions=Index vector (dialog)  Indices=[7 3 5]  OutputSizes=1  InputPortWidth=7  mask(Mux Selector (MBDLibrary)){InputPortWidth_mbdlib=7, Indices_mbdlib=[7 3 5]}
      mask prompts: InputPortWidth_mbdlib "Input Port Width"; Indices_mbdlib "Output Indices"
      mask help: Changes the order of the inputs.
      settings: OpenFcn=|
      | if exist('mbdlib_dialog')
      |    mbdlib_dialog(gcb,'open')
      | else
      |    open_system(gcb, 'mask')
      | end
      settings: CloseFcn=|
      | if exist('mbdlib_selector')
      |    mbdlib_selector(gcb)
      | end
      mask Help: The SELECTOR block is a MULTIPLEXED SELECTOR block, used to change the input/output order of a multiplexed data stream.
      mask Display:
      | port_label('input', 1,'[7]')
      | text(1.0,0.83333,'7', 'horizontalAlignment', 'right')
      | text(1.0,0.5,'3', 'horizontalAlignment', 'right')
      | text(1.0,0.16667,'5', 'horizontalAlignment', 'right')
  column2 : Selector  Tag=MBDLibrary v2007b.1  IndexOptions=Index vector (dialog)  Indices=[6 7 1]  OutputSizes=1  InputPortWidth=7  mask(Mux Selector (MBDLibrary)){InputPortWidth_mbdlib=7, Indices_mbdlib=[6 7 1]}
      mask prompts: InputPortWidth_mbdlib "Input Port Width"; Indices_mbdlib "Output Indices"
      mask help: Changes the order of the inputs.
      settings: OpenFcn=|
      | if exist('mbdlib_dialog')
      |    mbdlib_dialog(gcb,'open')
      | else
      |    open_system(gcb, 'mask')
      | end
      settings: CloseFcn=|
      | if exist('mbdlib_selector')
      |    mbdlib_selector(gcb)
      | end
      mask Help: The SELECTOR block is a MULTIPLEXED SELECTOR block, used to change the input/output order of a multiplexed data stream.
      mask Display:
      | port_label('input', 1,'[7]')
      | text(1.0,0.83333,'6', 'horizontalAlignment', 'right')
      | text(1.0,0.5,'7', 'horizontalAlignment', 'right')
      | text(1.0,0.16667,'1', 'horizontalAlignment', 'right')
  column3 : Selector  Tag=MBDLibrary v2007b.1  IndexOptions=Index vector (dialog)  Indices=[2 4 7]  OutputSizes=1  InputPortWidth=7  mask(Mux Selector (MBDLibrary)){InputPortWidth_mbdlib=7, Indices_mbdlib=[2 4 7]}
      mask prompts: InputPortWidth_mbdlib "Input Port Width"; Indices_mbdlib "Output Indices"
      mask help: Changes the order of the inputs.
      settings: OpenFcn=|
      | if exist('mbdlib_dialog')
      |    mbdlib_dialog(gcb,'open')
      | else
      |    open_system(gcb, 'mask')
      | end
      settings: CloseFcn=|
      | if exist('mbdlib_selector')
      |    mbdlib_selector(gcb)
      | end
      mask Help: The SELECTOR block is a MULTIPLEXED SELECTOR block, used to change the input/output order of a multiplexed data stream.
      mask Display:
      | port_label('input', 1,'[7]')
      | text(1.0,0.83333,'2', 'horizontalAlignment', 'right')
      | text(1.0,0.5,'4', 'horizontalAlignment', 'right')
      | text(1.0,0.16667,'7', 'horizontalAlignment', 'right')
  matrixConcat : Concatenate  Tag=MBDLibrary v2007b.1  NumInputs=3  Mode=Multidimensional array  ConcatenateDimension=2  mask(Matrix Concat (MBDLibrary)){concatDim=Horizontal, numInputs_mbdlib=3}
      mask prompts: concatDim "Type of Concatenate"; numInputs_mbdlib "Number of Inputs"
      mask help: Concatenate input signals of the same data type to create a contiguous output signal.
      settings: OpenFcn=|
      | if exist('mbdlib_dialog')
      |    mbdlib_dialog(gcb,'open')
      | else
      |    open_system(gcb, 'mask')
      | end
      settings: CloseFcn=|
      | if exist('mbdlib_matrixConcatenate')
      |    mbdlib_matrixConcatenate(gcb, 'mask')
      | end
      mask Help:
      | The MATRIX CONCAT block concatenates input signals from the dame data type and creates a contigouos output matrix.
      | In vector mode, all input signals must be either vectors or one-row [1xM] matrices or one-column [Mx1] matrices or a combination of vectors and either one-row matrices or one-column matrices. The output is a vector if all inputs are vectors. The output is a one-row or one-column matrix if any of the inputs are one-row or one-column matrices respectively.
      | 
      | Matrix mode treats vector inputs as one-column matrices. The output is always a matrix.
      mask StyleString: popup(Vertical|Horizontal),edit
      mask Display:
      | plot([0.1 0.3 0.3 0.1 0.1], [0.1 0.1 0.9 0.9 0.1])
      | plot([0.4 0.6 0.6 0.4 0.4], [0.1 0.1 0.9 0.9 0.1])
      | plot([0.7 0.9 0.9 0.7 0.7], [0.1 0.1 0.9 0.9 0.1])
  mux : Mux  Tag=MBDLibrary v2007b.1  Inputs=3  mask(Mux (MBDLibrary)){Inputs_mbdlib=3}
      mask prompts: Inputs_mbdlib "Number of Inputs"
      mask help: Converts multipule inputs to a vector.
      settings: OpenFcn=|
      | if exist('mbdlib_dialog')
      |    mbdlib_dialog(gcb,'open')
      | else
      |    open_system(gcb, 'mask')
      | end
      mask Help: The MUX block provides a vector output to the model for separate inputs.  The output order will correspond to the input order (from the first input at the top of the block to the last input at the bottom of the block).
  negative : Gain  Tag=MBDLibrary v2007b.1  Gain=-1  ParameterDataType=fixdt(1,16,0)  ParameterScaling=[]  OutDataType=fixdt(1,16,0)  OutScaling=[]  RndMeth=Zero  mask(Gain (MBDLibrary)){gain_mbdlib=-1}
      mask prompts: gain_mbdlib "Gain"
      mask help: Multiplies the input by the gain.
      settings: OpenFcn=|
      | if exist('mbdlib_dialog')
      |    mbdlib_dialog(gcb,'open')
      | else
      |    open_system(gcb, 'mask')
      | end
      mask Help: The GAIN block multiplies the input by the gain value.  This block may accept any data types other than boolean.  The user must take care to not use a non-integer gain for int32/uint32 inputs.
      mask Display: disp([get_param(gcb, 'Gain') 'x'])
  zero : Constant  Tag=MBDLibrary v2007b.1  Value=0  VectorParams1D=off  OutDataType=fixdt(1,16,0)  OutScaling=[]  mask(Constant (MBDLibrary)){Value_mbdlib=0, OutDataTypeMode_mbdlib=double}
      mask prompts: Value_mbdlib "Constant"; OutDataTypeMode_mbdlib "Data Type"
      mask help: Outputs a constant value
      settings: AttributesFormatString={%<OutDataTypeMode>}
      settings: OpenFcn=|
      | if exist('mbdlib_dialog')
      |    mbdlib_dialog(gcb,'open')
      | else
      |    open_system(gcb, 'mask')
      | end
      settings: CloseFcn=|
      | if exist('mbdlib_dialog')
      |    mbdlib_constant(gcb)
      | end
      mask Help: The CONSTANT block outputs a constant value to the system.
      mask StyleString: edit,popup(double|single|boolean|int32|uint32)
  skewLibOut : Outport  OutDataType=fixdt(1,16,0)  OutScaling=[]
  wires:
  zero/1 -> mux/3
  negative/1 -> mux/2
  column3/1 -> matrixConcat/3
  column2/1 -> matrixConcat/2
  column1/1 -> matrixConcat/1
  matrixConcat/1 -> skewLibOut/1
  mux/1 -> column1/1, column3/1, column2/1
  skewLibIn/1 -> mux/1, negative/1
